simulink model "closed_loop"  (R2020a)
settings: Solver=VariableStepAuto  StartTime=0.0  StopTime=50  RelTol=1e-3
undefined symbols (not defined in the file): C1, C2, ctrl_z, inner_h, omega_max_lim, omega_min_lim, sample_time, y_ref
libraries: simulink x1
settings Model: Creator=martinhe  LastModifiedBy=martinhe

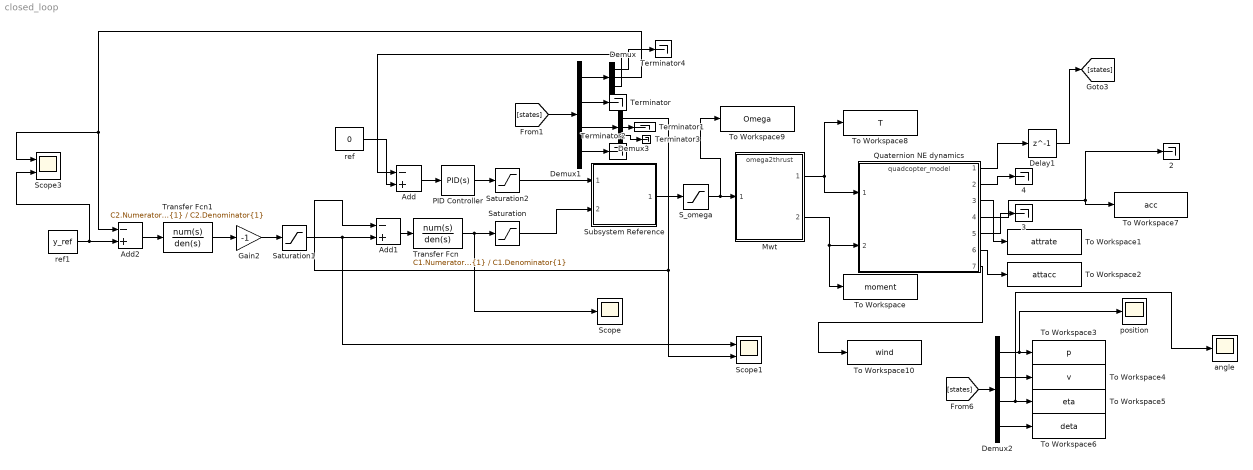
== system closed_loop ==
  "   2" : Terminator
  "   3" : Terminator
  "   4" : Terminator
  Add : Sum  Inputs=-+
  Add1 : Sum  Inputs=-+
  Add2 : Sum  Inputs=-+
  Delay1 : Delay  DelayLength=1  SampleTime=inner_h
  Demux : Demux  Outputs=3
  Demux1 : Demux  Outputs=[3,3,3,3]
  Demux2 : Demux  Outputs=[3,3,3,3]
  Demux3 : Demux  Outputs=3
  Gain2 : Gain  Gain=-1
  Mwt : ModelReference  ModelNameDialog=omega2thrust.mdl  SimulationMode=Normal  ModelReferenceVersion=1.5
  PID Controller : simulink/Continuous/PID Controller  Controller=PID  Form=Parallel  TimeDomain=Continuous-time  UseExternalTs=off  SampleTime=-1  IntegratorMethod=Forward Euler  FilterMethod=Forward Euler  ControllerParametersSource=internal  P=ctrl_z.Kp  I=ctrl_z.Ki  D=ctrl_z.Kd  UseFilter=on  N=100  TunerSelectOption=Transfer Function Based (PID Tuner App)  InitialConditionSource=internal  InitialConditionForIntegrator=0  InitialConditionForFilter=0  DifferentiatorICPrevScaledInput=0  ExternalReset=none  TrackingMode=off  Kt=1  LimitOutput=off  UpperSaturationLimit=inf  LowerSaturationLimit=-inf  LinearizeAsGain=on  AntiWindupMode=none  Kb=1  POutMin=[]  POutMax=[]  IOutMin=[]  IOutMax=[]  DOutMin=[]  DOutMax=[]  NOutMin=[]  NOutMax=[]  SumOutMin=[]  SumOutMax=[]  SaturationOutMin=[]  SaturationOutMax=[]  PParamMin=[]  PParamMax=[]  IParamMin=[]  IParamMax=[]  DParamMin=[]  DParamMax=[]  NParamMin=[]  NParamMax=[]  KbParamMin=[]  KbParamMax=[]  KtParamMin=[]  KtParamMax=[]  KbOutMin=[]  KbOutMax=[]  KtOutMin=[]  KtOutMax=[]  IntegratorOutMin=[]  IntegratorOutMax=[]  FilterOutMin=[]  FilterOutMax=[]  SumI1OutMin=[]  SumI1OutMax=[]  SumI2OutMin=[]  SumI2OutMax=[]  SumI3OutMin=[]  SumI3OutMax=[]  SumI4OutMin=[]  SumI4OutMax=[]  SumDOutMin=[]  SumDOutMax=[]  DifferentiatorOutMin=[]  DifferentiatorOutMax=[]  FilterDiffOutCoefMin=[]  FilterDiffOutCoefMax=[]  ReciprocalOutMin=[]  ReciprocalOutMax=[]  SumDenOutMin=[]  SumDenOutMax=[]  SumNumOutMin=[]  SumNumOutMax=[]  DivideOutMin=[]  DivideOutMax=[]  UdiffTsProdOutMin=[]  UdiffTsProdOutMax=[]  NTsProdOutMin=[]  NTsProdOutMax=[]  UintegralTsProdOutMin=[]  UintegralTsProdOutMax=[]  UngainTsProdOutMin=[]  UngainTsProdOutMax=[]  IntegratorContinuousStateAttributes=''  IntegratorStateMustResolveToSignalObject=off  IntegratorRTWStateStorageClass=Auto  FilterContinuousStateAttributes=''  FilterStateMustResolveToSignalObject=off  FilterRTWStateStorageClass=Auto  ParallelPVariant=InternalParameters  IdealPVariant=Disabled  IVariant=InternalParameters  DVariant=InternalParameters  IntegratorVariant=Continuous  SatVariant=Disabled  AWVariant=Passthrough  PCopyVariant=Disabled  TRVariant=Disabled  FdbkBlocksVariant=Forward  IdealPFdbkVariant=Disabled  SatFdbkVariant=Disabled  DerivativeFilterVariant=ContFilter  NVariant=InternalParameters  NCopyVariant=Disabled  FilterICVariant=InternalICsFilter  IntegratorICVariant=InternalICs  ExternalResetVariant=Disabled  TRSumVariant=Passthrough  SumFdbkVariant=Disabled  SumVariant=Sum_PID  TsampFilterVariant=InternalTs  TsampNgainVariant=Passthrough  TsampIntegralVariant=Passthrough
  Quaternion NE dynamics : ModelReference  ModelNameDialog=quadcopter_model.mdl  SimulationMode=Normal  ModelReferenceVersion=1.342
  S_omega : Saturate  UpperLimit=omega_max_lim  LowerLimit=omega_min_lim
  Saturation : Saturate  UpperLimit=1e-3  LowerLimit=-1e-3
  Saturation1 : Saturate  UpperLimit=pi/15  LowerLimit=-pi/15
  Saturation2 : Saturate  UpperLimit=inf  LowerLimit=-inf
  Scope : Scope
  Scope1 : Scope  NumInputPorts=2
  Scope3 : Scope  NumInputPorts=2
  Subsystem Reference : Subsystem  ReferencedSubsystem=thrust2omega
  Terminator{,1..4} (5 alike) : Terminator
  To Workspace : ToWorkspace  VariableName=moment  SaveFormat=Timeseries  SampleTime=sample_time
  To Workspace1 : ToWorkspace  VariableName=attrate  SaveFormat=Timeseries  SampleTime=sample_time
  To Workspace10 : ToWorkspace  VariableName=wind  SaveFormat=Timeseries  SampleTime=sample_time
  To Workspace2 : ToWorkspace  VariableName=attacc  SaveFormat=Timeseries  SampleTime=sample_time
  To Workspace3 : ToWorkspace  VariableName=p  SaveFormat=Timeseries  SampleTime=sample_time
  To Workspace4 : ToWorkspace  VariableName=v  SaveFormat=Timeseries  SampleTime=sample_time
  To Workspace5 : ToWorkspace  VariableName=eta  SaveFormat=Timeseries  SampleTime=sample_time
  To Workspace6 : ToWorkspace  VariableName=deta  SaveFormat=Timeseries  SampleTime=sample_time
  To Workspace7 : ToWorkspace  VariableName=acc  SaveFormat=Timeseries  SampleTime=sample_time
  To Workspace8 : ToWorkspace  VariableName=T  SaveFormat=Timeseries  SampleTime=sample_time
  To Workspace9 : ToWorkspace  VariableName=Omega  SaveFormat=Timeseries  SampleTime=sample_time
  Transfer Fcn : TransferFcn  Numerator=C1.Numerator{1}  Denominator=C1.Denominator{1}
  Transfer Fcn1 : TransferFcn  Numerator=C2.Numerator{1}  Denominator=C2.Denominator{1}
  angle : Scope
  position : Scope
  ref : Constant  Value=0
  ref1 : Constant  Value=y_ref
  wires:
  Quaternion NE dynamics/5 -> "   3"/1
  Quaternion NE dynamics/3 -> To Workspace1/1
  Quaternion NE dynamics/6 -> To Workspace2/1
  [states] -> Demux2/1
  Demux2/2 -> To Workspace4/1
  Demux2/3 -> angle/1, To Workspace5/1
  Quaternion NE dynamics/4 -> "   2"/1, To Workspace7/1
  Mwt/1 -> To Workspace8/1, Quaternion NE dynamics/1
  Demux2/1 -> position/1, To Workspace3/1
  S_omega/1 -> To Workspace9/1, Mwt/1
  Quaternion NE dynamics/2 -> "   4"/1
  Mwt/2 -> To Workspace/1, Quaternion NE dynamics/2
  Demux2/4 -> To Workspace6/1
  [states] -> Demux1/1
  Demux1/1 -> Demux/1
  Demux1/2 -> Terminator/1
  Demux1/3 -> Demux3/1
  Demux1/4 -> Terminator2/1
  Subsystem Reference/1 -> S_omega/1
  ref/1 -> Add/2
  Add/1 -> PID Controller/1
  Demux/1 -> Terminator4/1
  Demux/3 -> Add/1
  Transfer Fcn/1 -> Scope/1, Saturation/1
  Add2/1 -> Transfer Fcn1/1
  ref1/1 -> Scope3/2, Add2/2
  Demux/2 -> Add2/1, Scope3/1
  PID Controller/1 -> Saturation2/1
  Saturation1/1 -> Scope1/1, Add1/2
  Quaternion NE dynamics/7 -> To Workspace10/1
  Add1/1 -> Transfer Fcn/1
  Demux3/1 -> Add1/1, Scope1/2
  Transfer Fcn1/1 -> Gain2/1
  Gain2/1 -> Saturation1/1
  Saturation2/1 -> Subsystem Reference/1
  Saturation/1 -> Subsystem Reference/2
  Demux3/2 -> Terminator1/1
  Demux3/3 -> Terminator3/1
  Quaternion NE dynamics/1 -> Delay1/1
  Delay1/1 -> [states]
